simulink library "cbobsv2p5"  (Simulink 5.0)
values from neighbouring files (symbols this model uses):
  b = findobj(a, 'Name', get_param(gcbh,'Name'))    [eyediasi2.m]
undefined symbols (not defined in the file or in its folder): eyediasi2, remez
libraries: commblksprivate x14, dspsigattribs x10, dspmlti3 x6, simulink3 x6, dspsrcs4 x4, commsrccod2 x2, dsparch3 x1
settings Model: Creator=mmclerno  LastModifiedBy=mclune  ExtModeAutoUpdateStatusClock=off

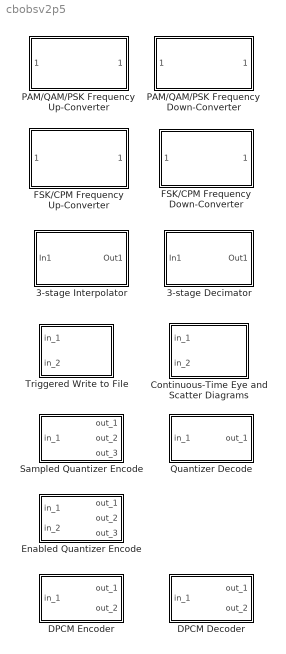
== system cbobsv2p5 ==
  3-stage Decimator : Subsystem  mask(3-stage Decimator){decFactor=10, Tin=1/10000, Fmax=450}
      mask prompts: decFactor "Decimation factor:"; Tin "Input sample time (s):"; Fmax "Maximum signal frequency (Hz):"
      mask help:
      | Performs decimation on the input signal.  The block uses multi-stage FIR filtering to eliminate aliasing, because using multiple stages is more efficient than using a single stage.
      |
      | For most efficient results, large decimation factors should have at least three factors.
      mask init:
      | dec_params = commblkdecimtr(gcb,'init');
      mask Display: disp('3-stage\nDecimator')
  3-stage Interpolator : Subsystem  mask(3-stage Interpolator){intFactor=10, Tin=1/1000, Fmax=450}
      mask prompts: intFactor "Interpolation factor:"; Tin "Input sample time (s):"; Fmax "Maximum signal frequency (Hz):"
      mask help:
      | Performs a interpolation on the input signal.  The block uses multi-stage FIR filtering to eliminate spectral copies because using multiple stages is more efficient than using a single stage.
      |
      | For most efficient results, large interpolation factors should have at least three factors.
      mask init:
      | int_params = commblkintrpltr(gcb,'init');
      mask Display: disp('3-stage\n Interpolator')
  Continuous-Time Eye and Scatter Diagrams : Subsystem  LoadFcn=eyediasi2([],[],[],'LoadBlock')  StartFcn=eyediasi2([],[],[],'Start')  StopFcn=eyediasi2([],[],[],'Stop')  mask(Continuous-Time Eye and Scatter Diagrams){time_range=1, time_offset=0, boundary=[-1.5 1.5], kept_length=5, diagram_type=Eye Diagram, eye_line=b-/r-, scatter_line=b., two_d_line=b-}
      mask prompts: time_range "Trace period:"; time_offset "Trace offset:"; boundary "Lower and upper bounds of diagram (2-element vector):"; kept_length "Number of saved traces:"; diagram_type "Diagram type:"; eye_line "Line type for eye diagram:"; scatter_line "Line type for scatter diagram:"; two_d_line "Line type for X-Y diagram:"
      mask help: Create an eye diagram with or without a scatter diagram or an X-Y diagram depending on Diagram type parameter. Use the trigger input to determine the decision time for the scatter plot.
      mask init:
      | [a,b]=trigicon(0,25,get_param(gcb,'orientation'),2);
      | x = [2 8 5 2 8 5 5 5];
      | y = [2 8 5 8 2 5 8 2];
      | [eStr outparams] = commblkeyescatcont(gcb,'init');
      | if(eStr .ecode ~= 0)
      |    error(eStr .emsg);
      | end
      settings: CopyFcn=eyediasi2([],[],[],'CopyBlock')  DeleteFcn=eyediasi2([],[],[],'DeleteBlock')  NameChangeFcn=eyediasi2([],[],[],'NameChange')
      mask Help: helpview(commbhelp)
      mask StyleString: edit,edit,edit,edit,popup(Eye Diagram|Scatter Diagram|Eye and Scatter Diagrams|X-Y Diagram|Eye and X-Y Diagrams),edit,edit,edit
      mask CallbackString: ||||commblkeyescatcont(gcb,'cbDiagram_type');|||
      mask Display: plot(0,0,100,100,[5 45 45 5 5 5 5+40*[0:1/15:1] 5+40*[1:-1/15:0] 5+40*[0:1/15:1] 5+40*[1:-1/15:0]], [35 35 95 95 35 65 sin([0:1/15:1]*pi)*25+65 sin(-[0:1/15:1]*pi)*25+65 sin([0:1/15:1]*pi)*17+65 sin(-[0:1/15:1]*pi)*18+65]*.95+3 ,a,b, NaN, NaN, x+50,y+37,x+50,y+52,x+50,y+67,x+50,y+82, x+62,y+37,x+62,y+52,x+62,y+67,x+62,y+82, x+73,y+37,x+73,y+52,x+73,y+67,x+73,y+82, x+85,y+37,x+85,y+52,x+85,y+67,x+85,y+82, [50 95 73 73 73],[65 65 65 35 95])
  DPCM Decoder : Subsystem  mask(DPCM Decoder){num=[0 .9963], den=1, codebook=[-.0848 -.029 .0298 .0853], sample_time=.1}
      mask prompts: num "Predictor numerator:"; den "Predictor denominator:"; codebook "Quantization codebook:"; sample_time "Sample time:"
      mask help:
      | Input the DPCM coded index. Output DPCM decodes to the 1st outport and quantization decode to the 2nd outport.
      |
      | The input must be a scalar signal.
      mask Help: helpview(commbhelp)
      mask Display: disp('DPCM\ndecoder')
  DPCM Encoder : Subsystem  mask(DPCM Encoder){num=[0 .9963], den=1, partition=[-.0569 .0004 .0576], codebook=[-.0848 -.029 .0298 .0853], sample_time=.1}
      mask prompts: num "Predictor numerator:"; den "Predictor denominator:"; partition "Quantization partition:"; codebook "Quantization codebook:"; sample_time "Sample time:"
      mask help:
      | Output the DPCM encoded index to the 1st outport and the quantization recovered value to the 2nd outport.
      |
      | The input must be a scalar signal.
      mask Help: helpview(commbhelp)
      mask Display: disp('DPCM\nencoder')
  Enabled Quantizer Encode : Subsystem  mask(Enabled Quantizer Encode){partition=[-.75 -.25 .25 .75], codebook=[-.825 -.5 0 .5 .825], n=2}
      mask prompts: partition "Quantization partition:"; codebook "Quantization codebook:"; n "Input signal vector length:"
      mask help:
      | Triggered by the 2nd input signal, this block quantizes an analog signal to (1) digital signal, (2) quantization value, and (3) distortion.
      |
      | The first input can be either a scalar, a sample-based vector, or a frame-based row vector.  Each vector element is processed independently.
      |
      | The trigger input must be a scalar.
      mask init:
      | [x,y]=trigicon(0,25,get_param(gcb,'orientation'),1);
      mask Help: helpview(commbhelp)
      mask Display: plot(0,0,100,100,x,y);disp('Quantizer')
  FSK/CPM Frequency Down-Converter : Subsystem  mask(FSK/CPM Frequency Down-Converter){modType=FSK, M=8, freqSep=100, td=1/100, Fc=3000, Ph=0, Tin=1/10000, Tout=1/1000}
      mask prompts: modType "Modulation type:"; M "M-ary number:"; freqSep "Frequency separation (Hz):"; td "Symbol period (s):"; Fc "Carrier frequency (Hz):"; Ph "Carrier phase (rad):"; Tin "Input sample time (s):"; Tout "Output sample time (s):"
      mask help:
      | The FSK/CPM Frequency Down-Converter translates the frequency of the passband input signal to complex baseband.  It also decimates the signal in order to prevent aliasing.
      |
      | The input signal must be a sample-based scalar.
      mask init:
      | Fmax = commblkfskdowncon(gcb,'init');
      mask StyleString: popup(FSK|CPM),edit,edit,edit,edit,edit,edit,edit
      mask CallbackString: commblkfskdowncon(gcb,'cbModType');|||||||
      mask Display: disp('FSK/CPM\nFrequency\nDown-Converter');
  FSK/CPM Frequency Up-Converter : Subsystem  mask(FSK/CPM Frequency Up-Converter){modType=FSK, M=8, freqSep=100, td=1/100, Fc=3000, Ph=0, Tin=1/1000, Tout=1/10000}
      mask prompts: modType "Modulation type:"; M "M-ary number:"; freqSep "Frequency separation (Hz):"; td "Symbol period (s):"; Fc "Carrier frequency (Hz):"; Ph "Carrier phase (rad):"; Tin "Input sample time (s):"; Tout "Output sample time (s):"
      mask help:
      | The FSK/CPM Frequency Up-Converter translates the frequency of the baseband input FSK or CPM signal to the carrier frequency.
      | It also interpolates the signal in order to prevent aliasing.
      |
      | The input signal must be a sample-based scalar.
      mask init:
      | Fmax = commblkfskupcon(gcb,'init');
      mask StyleString: popup(FSK|CPM),edit,edit,edit,edit,edit,edit,edit
      mask CallbackString: commblkfskupcon(gcb,'cbModType');|||||||
      mask Display: disp('FSK/CPM\nFrequency\nUp-Converter');
  PAM/QAM/PSK Frequency Down-Converter : Subsystem  mask(PAM/QAM/PSK Frequency Down-Converter){Fc=3000, Ph=0, Tin=1/8000, Tout=1/100}
      mask prompts: Fc "Carrier frequency (Hz):"; Ph "Carrier phase (rad):"; Tin "Input sample time:"; Tout "Output sample time:"
      mask help:
      | The PAM/QAM/PSK Frequency Down-Converter translates the frequency of the input signal to complex baseband.  It also decimates the signal to a lower sampling frequency.
      |
      | The input signal must be a sample-based scalar.
      mask init:
      | if (Tin>=1/(2*(Fc+1/Tout))) error('The reciprocal of the input sample time must be greater than twice the sum of the carrier frequency and the reciprocal of the output sample time.'); end;
      | 
      | if (Tout <= 1/Fc) error('The reciprocal of the output sample time must be less than the carrier frequency.'); end;
      | 
      | if (Tin>=Tout) error('The input sample time must be less than the output sample time.'); end;
      mask Display: disp('PAM/QAM/PSK\nFrequency\nDown-Converter');
  PAM/QAM/PSK Frequency Up-Converter : Subsystem  mask(PAM/QAM/PSK Frequency Up-Converter){Fc=3000, Ph=0, Tin=1/100, Tout=1/8000}
      mask prompts: Fc "Carrier frequency (Hz):"; Ph "Carrier phase (rad):"; Tin "Input sample time:"; Tout "Output sample time:"
      mask help:
      | The PAM/QAM/PSK Frequency Up-Converter translates the frequency of the baseband input signal to the carrier frequency.  It also resamples the signal to a higher sampling frequency.
      |
      | The input signal must be a sample-based scalar.
      mask init:
      | if (Tout>=1/(2*(Fc+1/Tin))) error('The reciprocal of the output sample time must be greater than twice the sum of the carrier frequency and the reciprocal of the input sample time.'); end;
      | 
      | if (Tin <= 1/Fc) error('The reciprocal of the input sample time must be less than the carrier frequency.'); end;
      | 
      | if (Tin<=Tout) error('The input sample time must be greater than the output sample time.'); end;
      mask Display: disp('PAM/QAM/PSK\nFrequency\nUp-Converter');
  Quantizer Decode : Subsystem  mask(Quantizer Decode){codebook=[-.825 -.5 0, .5 .825]}
      mask prompts: codebook "Quantization codebook:"
      mask help:
      | Output the value in the given codebook based on the input index value.
      |
      | The input can be either a scalar, a sample-based vector, or a frame-based row vector.  This block processes each vector element independently.
      mask Help: helpview(commbhelp)
      mask Display: disp('Quantizer\ndecode')
  Sampled Quantizer Encode : Subsystem  mask(Sampled Quantizer Encode){partition=[-.75 -.25 .25 .75], codebook=[-.825 -.5 0 .5 .825], n=2, sample_time=.1}
      mask prompts: partition "Quantization partition:"; codebook "Quantization codebook:"; n "Input signal vector length:"; sample_time "Sample time:"
      mask help:
      | Quantize an analog signal to (1) digital signal, (2) quantization value, and (3) distortion at every sample time point.
      |
      | The input can be either a scalar, a sample-based vector, or a frame-based row vector.  This block processes each vector element independently.
      mask Help: helpview(commbhelp)
      mask Display: disp('Scalar\nquantizer')
  Triggered Write to File : Subsystem  mask(Triggered Write to File){filename='untitled.dat', datatype=ASCII, dec=1, threshold=0.5}
      mask prompts: filename "File name (string, include extension):"; datatype "Data type:"; dec "Decimation:"; threshold "Threshold in detecting trigger signal:"
      mask help:
      | The rising edge of the signal from the 2nd port triggers the block to write another row into the specified file.
      |
      | Inputs must be sample-based.
      mask init:
      | [x,y]=trigicon(0,25,get_param(gcb,'orientation'),2);
      | nump = dec - 1;
      mask Help: helpview(commbhelp)
      mask StyleString: edit,popup(ASCII|binary|float|integer),edit,edit
      mask Display:
      | plot(0,0,100,100,100-[25 25 05 05 25 25 05 13 13 17 17 17 15 real(exp(j*pi*([0:20]/10+1/2)))*3.5+15 15 25 25 25+[0:1/30:1]*70],
      | [85 95 95 75 75 89 89 89 95 95 89 89 89 imag(exp(j*pi*([0:20]/10+1/2)))*3.5+85 89 89 85 -sin([0:1/30:1]*pi*2)*10+85]-15, x,y);disp('\n  Wt file')

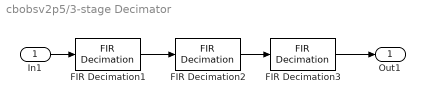
== system cbobsv2p5/3-stage Decimator ==
  In1 : Inport
  FIR Decimation1 : dspmlti3/FIR Decimation  h=remez(dec_params.order1, [0 dec_params.Fpass1 dec_params.Fstop1 1], [1 1 0 0])  D=dec_params.decFact1  framing=Maintain input frame size  outputBufInitCond=0
  FIR Decimation2 : dspmlti3/FIR Decimation  h=remez(dec_params.order2, [0 dec_params.Fpass2 dec_params.Fstop2 1], [1 1 0 0])  D=dec_params.decFact2  framing=Maintain input frame size  outputBufInitCond=0
  FIR Decimation3 : dspmlti3/FIR Decimation  h=remez(dec_params.order3, [0 dec_params.Fpass3 dec_params.Fstop3 1], [1 1 0 0])  D=dec_params.decFact3  framing=Maintain input frame size  outputBufInitCond=0
  Out1 : Outport
  wires:
  FIR Decimation1/1 -> FIR Decimation2/1
  FIR Decimation2/1 -> FIR Decimation3/1
  FIR Decimation3/1 -> Out1/1
  In1/1 -> FIR Decimation1/1

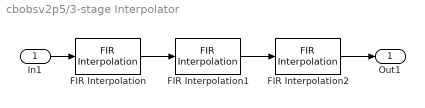
== system cbobsv2p5/3-stage Interpolator ==
  In1 : Inport
  FIR Interpolation : dspmlti3/FIR Interpolation  h=remez(int_params.order1, [0 int_params.Fpass1 int_params.Fstop1 1], [1 1 0 0]) * int_params.intFact1  L=int_params.intFact1  framing=Maintain input frame size  outputBufInitCond=0
  FIR Interpolation1 : dspmlti3/FIR Interpolation  h=remez(int_params.order2, [0 int_params.Fpass2 int_params.Fstop2 1], [1 1 0 0]) * int_params.intFact2  L=int_params.intFact2  framing=Maintain input frame size  outputBufInitCond=0
  FIR Interpolation2 : dspmlti3/FIR Interpolation  h=remez(int_params.order3, [0 int_params.Fpass3 int_params.Fstop3 1], [1 1 0 0]) * int_params.intFact3  L=int_params.intFact3  framing=Maintain input frame size  outputBufInitCond=0
  Out1 : Outport
  wires:
  FIR Interpolation2/1 -> Out1/1
  FIR Interpolation1/1 -> FIR Interpolation2/1
  FIR Interpolation/1 -> FIR Interpolation1/1
  In1/1 -> FIR Interpolation/1

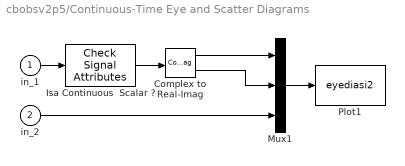
== system cbobsv2p5/Continuous-Time Eye and Scatter Diagrams ==
  in_1 : Inport
  in_2 : Inport  Port=2
  Complex to Real-Imag : ComplexToRealImag
  Isa Continuous  Scalar ? : dspsigattribs/Check Signal Attributes  SigAttribCheckMethod=Does not match attributes exactly  Complexity=Ignore  Frame=Sample-based  DimsCheckMethod=Is...  Dimensions=Scalar (1-D or 2-D)  DatatypeCheckMethod=Is not...  DatatypeGeneral=Boolean  DtypeFloatSpecific=Any floating-point  DtypeFixedSpecific=Any fixed-point  DtypeIntSpecific=Any integer  SampleMode=Continuous
  Mux1 : Mux  Inputs=3
  Plot1 : S-Function  FunctionName=eyediasi2  Parameters=time_range, time_offset, boundary, kept_length, diagram_type, eye_line, scatter_line, two_d_line
  wires:
  in_2/1 -> Mux1/3
  in_1/1 -> Isa Continuous  Scalar ?/1
  Complex to Real-Imag/2 -> Mux1/2
  Complex to Real-Imag/1 -> Mux1/1
  Mux1/1 -> Plot1/1
  Isa Continuous  Scalar ?/1 -> Complex to Real-Imag/1

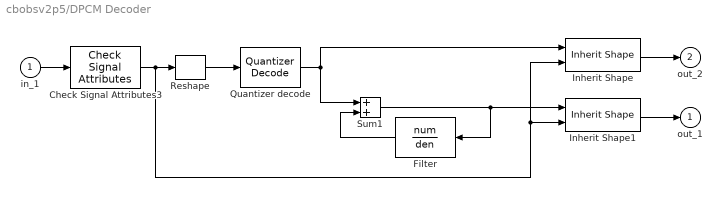
== system cbobsv2p5/DPCM Decoder ==
  in_1 : Inport
  Check Signal Attributes3 : dspsigattribs/Check Signal Attributes  SigAttribCheckMethod=Does not match attributes exactly  Complexity=Ignore  Frame=Ignore  DimsCheckMethod=Is...  Dimensions=Scalar (1-D or 2-D)  DatatypeCheckMethod=Ignore  DatatypeGeneral=Boolean  DtypeFloatSpecific=Any floating-point  DtypeFixedSpecific=Any fixed-point  DtypeIntSpecific=Any integer  SampleMode=Ignore
  Filter : DiscreteFilter  Orientation=left  Numerator=num  Denominator=den  SampleTime=sample_time
  Inherit Shape : commblksprivate/Inherit Shape
  Inherit Shape1 : commblksprivate/Inherit Shape
  Quantizer decode : commsrccod2/Quantizer Decode  codebook=codebook
  Reshape : simulink3/Signals & Systems/Reshape  OutputDimensionality=1-D array  OutputDimensions=[1,1]
  Sum1 : Sum  SaturateOnIntegerOverflow=on  InputSameDT=on
  out_1 : Outport  InitialOutput=0
  out_2 : Outport  Port=2  InitialOutput=0
  wires:
  Inherit Shape1/1 -> out_1/1
  Inherit Shape/1 -> out_2/1
  Reshape/1 -> Quantizer decode/1
  Check Signal Attributes3/1 -> Inherit Shape/2, Inherit Shape1/2, Reshape/1
  in_1/1 -> Check Signal Attributes3/1
  Filter/1 -> Sum1/2
  Sum1/1 -> Inherit Shape1/1, Filter/1
  Quantizer decode/1 -> Inherit Shape/1, Sum1/1

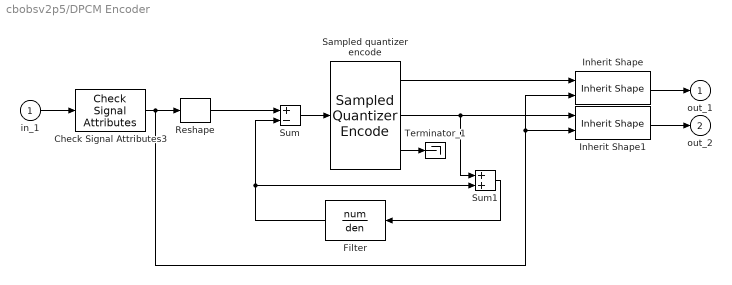
== system cbobsv2p5/DPCM Encoder ==
  in_1 : Inport
  Check Signal Attributes3 : dspsigattribs/Check Signal Attributes  SigAttribCheckMethod=Does not match attributes exactly  Complexity=Ignore  Frame=Ignore  DimsCheckMethod=Is...  Dimensions=Scalar (1-D or 2-D)  DatatypeCheckMethod=Ignore  DatatypeGeneral=Boolean  DtypeFloatSpecific=Any floating-point  DtypeFixedSpecific=Any fixed-point  DtypeIntSpecific=Any integer  SampleMode=Ignore
  Filter : DiscreteFilter  Orientation=left  Numerator=num  Denominator=den  SampleTime=sample_time
  Inherit Shape : commblksprivate/Inherit Shape
  Inherit Shape1 : commblksprivate/Inherit Shape
  Reshape : simulink3/Signals & Systems/Reshape  OutputDimensionality=1-D array  OutputDimensions=[1,1]
  Sampled quantizer encode : commsrccod2/Sampled Quantizer Encode  partition=partition  codebook=codebook  n=1  sample_time=sample_time
  Sum : Sum  Inputs=+-  SaturateOnIntegerOverflow=on  InputSameDT=on
  Sum1 : Sum  SaturateOnIntegerOverflow=on  InputSameDT=on
  Terminator_1 : Terminator
  out_1 : Outport  InitialOutput=0
  out_2 : Outport  Port=2  InitialOutput=0
  wires:
  Inherit Shape1/1 -> out_2/1
  Inherit Shape/1 -> out_1/1
  Sampled quantizer encode/1 -> Inherit Shape/1
  Reshape/1 -> Sum/1
  Check Signal Attributes3/1 -> Inherit Shape1/2, Inherit Shape/2, Reshape/1
  Sum1/1 -> Filter/1
  Filter/1 -> Sum/2, Sum1/2
  in_1/1 -> Check Signal Attributes3/1
  Sum/1 -> Sampled quantizer encode/1
  Sampled quantizer encode/2 -> Inherit Shape1/1, Sum1/1
  Sampled quantizer encode/3 -> Terminator_1/1

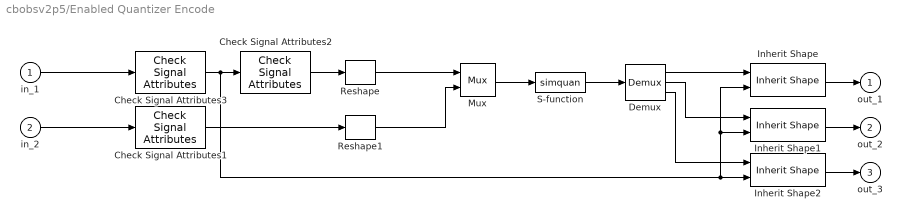
== system cbobsv2p5/Enabled Quantizer Encode ==
  in_1 : Inport
  in_2 : Inport  Port=2
  Check Signal Attributes1 : dspsigattribs/Check Signal Attributes  SigAttribCheckMethod=Does not match attributes exactly  Complexity=Ignore  Frame=Ignore  DimsCheckMethod=Is...  Dimensions=Scalar (1-D or 2-D)  DatatypeCheckMethod=Ignore  DatatypeGeneral=Boolean  DtypeFloatSpecific=Any floating-point  DtypeFixedSpecific=Any fixed-point  DtypeIntSpecific=Any integer  SampleMode=Ignore
  Check Signal Attributes2 : dspsigattribs/Check Signal Attributes  SigAttribCheckMethod=Matches attributes exactly  Complexity=Ignore  Frame=Frame-based  DimsCheckMethod=Is...  Dimensions=Column vector (2-D)  DatatypeCheckMethod=Ignore  DatatypeGeneral=Boolean  DtypeFloatSpecific=Any floating-point  DtypeFixedSpecific=Any fixed-point  DtypeIntSpecific=Any integer  SampleMode=Ignore
  Check Signal Attributes3 : dspsigattribs/Check Signal Attributes  SigAttribCheckMethod=Matches attributes exactly  Complexity=Ignore  Frame=Ignore  DimsCheckMethod=Is...  Dimensions=Full matrix (2-D)  DatatypeCheckMethod=Ignore  DatatypeGeneral=Boolean  DtypeFloatSpecific=Any floating-point  DtypeFixedSpecific=Any fixed-point  DtypeIntSpecific=Any integer  SampleMode=Ignore
  Demux : Demux  Outputs=[n n n]
  Inherit Shape : commblksprivate/Inherit Shape
  Inherit Shape1 : commblksprivate/Inherit Shape
  Inherit Shape2 : commblksprivate/Inherit Shape
  Mux : Mux  Inputs=[n 1]
  Reshape : simulink3/Signals & Systems/Reshape  OutputDimensionality=1-D array  OutputDimensions=[1,1]
  Reshape1 : simulink3/Signals & Systems/Reshape  OutputDimensionality=1-D array  OutputDimensions=[1,1]
  S-function : S-Function  FunctionName=simquan  Parameters=n, partition, codebook
  out_1 : Outport  InitialOutput=0
  out_2 : Outport  Port=2  InitialOutput=0
  out_3 : Outport  Port=3  InitialOutput=0
  wires:
  Reshape1/1 -> Mux/2
  Reshape/1 -> Mux/1
  Check Signal Attributes2/1 -> Reshape/1
  Check Signal Attributes1/1 -> Reshape1/1
  Demux/3 -> Inherit Shape2/1
  Demux/2 -> Inherit Shape1/1
  Inherit Shape2/1 -> out_3/1
  Inherit Shape1/1 -> out_2/1
  Demux/1 -> Inherit Shape/1
  Inherit Shape/1 -> out_1/1
  Check Signal Attributes3/1 -> Inherit Shape1/2, Inherit Shape/2, Inherit Shape2/2, Check Signal Attributes2/1
  in_1/1 -> Check Signal Attributes3/1
  in_2/1 -> Check Signal Attributes1/1
  Mux/1 -> S-function/1
  S-function/1 -> Demux/1

== system cbobsv2p5/FSK/CPM Frequency Down-Converter ==
  " " : Inport  SampleTime=Tin
  3-stage Decimator : commblksprivate/3-stage Decimator  decFactor=Tout / Tin  Tin=Tin  Fmax=Fmax
  Complex Carrier : dspsrcs4/Sine Wave  Amplitude=sqrt(2)  Frequency=-Fc  Phase=-Ph  SampleMode=Discrete  OutComplex=Complex  CompMethod=Trigonometric fcn  TableSize=Speed  SampleTime=Tin  SamplesPerFrame=1  dType=Double  ResetState=Restart at time zero
  Product1 : Product  SaturateOnIntegerOverflow=on  InputSameDT=on
  "  " : Outport
  wires:
  Product1/1 -> 3-stage Decimator/1
  Complex Carrier/1 -> Product1/2
  " "/1 -> Product1/1
  3-stage Decimator/1 -> "  "/1

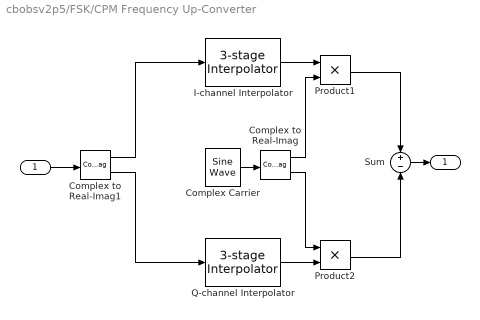
== system cbobsv2p5/FSK/CPM Frequency Up-Converter ==
  " " : Inport
  Complex Carrier : dspsrcs4/Sine Wave  Amplitude=sqrt(2)  Frequency=Fc  Phase=Ph  SampleMode=Discrete  OutComplex=Complex  CompMethod=Trigonometric fcn  TableSize=Speed  SampleTime=Tout  SamplesPerFrame=1  dType=Double  ResetState=Restart at time zero
  Complex to Real-Imag : ComplexToRealImag
  Complex to Real-Imag1 : ComplexToRealImag
  I-channel Interpolator : commblksprivate/3-stage Interpolator  intFactor=Tin / Tout  Tin=Tin  Fmax=Fmax
  Product1 : Product  SaturateOnIntegerOverflow=on  InputSameDT=on
  Product2 : Product  SaturateOnIntegerOverflow=on  InputSameDT=on
  Q-channel Interpolator : commblksprivate/3-stage Interpolator  intFactor=Tin / Tout  Tin=Tin  Fmax=Fmax
  Sum : Sum  Inputs=+|-  SaturateOnIntegerOverflow=on  InputSameDT=on
  "  " : Outport
  wires:
  Complex to Real-Imag1/1 -> I-channel Interpolator/1
  I-channel Interpolator/1 -> Product1/1
  Sum/1 -> "  "/1
  Product2/1 -> Sum/2
  Product1/1 -> Sum/1
  Complex to Real-Imag/2 -> Product2/1
  Complex to Real-Imag/1 -> Product1/2
  " "/1 -> Complex to Real-Imag1/1
  Complex Carrier/1 -> Complex to Real-Imag/1
  Q-channel Interpolator/1 -> Product2/2
  Complex to Real-Imag1/2 -> Q-channel Interpolator/1

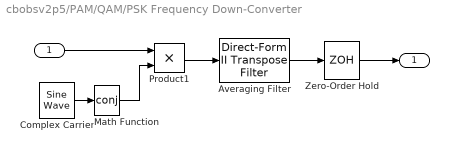
== system cbobsv2p5/PAM/QAM/PSK Frequency Down-Converter ==
  " " : Inport  SampleTime=Tin
  Averaging Filter : dsparch3/Direct-Form II Transpose Filter  num=(Tin/Tout)*ones(1,floor(Tout/Tin))  den=1  ic=0
  Complex Carrier : dspsrcs4/Sine Wave  Amplitude=sqrt(2)  Frequency=Fc  Phase=Ph  SampleMode=Discrete  OutComplex=Complex  CompMethod=Trigonometric fcn  TableSize=Speed  SampleTime=Tin  SamplesPerFrame=1  dType=Double  ResetState=Restart at time zero
  Math Function : Math  Operator=conj
  Product1 : Product  SaturateOnIntegerOverflow=on  InputSameDT=on
  Zero-Order Hold : ZeroOrderHold  SampleTime=Tout
  "  " : Outport
  wires:
  Averaging Filter/1 -> Zero-Order Hold/1
  Product1/1 -> Averaging Filter/1
  Complex Carrier/1 -> Math Function/1
  Math Function/1 -> Product1/2
  " "/1 -> Product1/1
  Zero-Order Hold/1 -> "  "/1

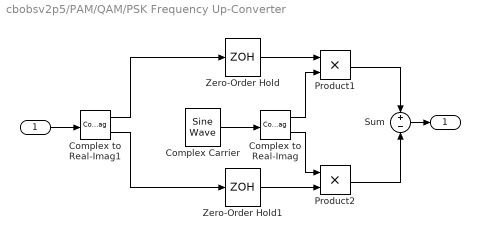
== system cbobsv2p5/PAM/QAM/PSK Frequency Up-Converter ==
  " " : Inport
  Complex Carrier : dspsrcs4/Sine Wave  Amplitude=sqrt(2)  Frequency=Fc  Phase=Ph  SampleMode=Discrete  OutComplex=Complex  CompMethod=Trigonometric fcn  TableSize=Speed  SampleTime=Tout  SamplesPerFrame=1  dType=Double  ResetState=Restart at time zero
  Complex to Real-Imag : ComplexToRealImag
  Complex to Real-Imag1 : ComplexToRealImag
  Product1 : Product  SaturateOnIntegerOverflow=on  InputSameDT=on
  Product2 : Product  SaturateOnIntegerOverflow=on  InputSameDT=on
  Sum : Sum  Inputs=+|-  SaturateOnIntegerOverflow=on  InputSameDT=on
  Zero-Order Hold : ZeroOrderHold  SampleTime=Tout
  Zero-Order Hold1 : ZeroOrderHold  SampleTime=Tout
  "  " : Outport
  wires:
  Complex Carrier/1 -> Complex to Real-Imag/1
  Sum/1 -> "  "/1
  Product2/1 -> Sum/2
  Product1/1 -> Sum/1
  Complex to Real-Imag/2 -> Product2/1
  Complex to Real-Imag/1 -> Product1/2
  Complex to Real-Imag1/1 -> Zero-Order Hold/1
  Complex to Real-Imag1/2 -> Zero-Order Hold1/1
  " "/1 -> Complex to Real-Imag1/1
  Zero-Order Hold/1 -> Product1/1
  Zero-Order Hold1/1 -> Product2/2

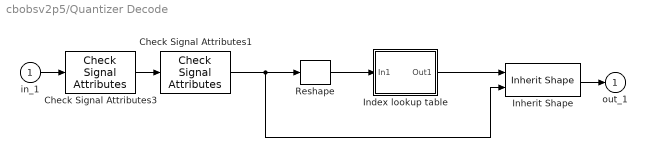
== system cbobsv2p5/Quantizer Decode ==
  in_1 : Inport
  Check Signal Attributes1 : dspsigattribs/Check Signal Attributes  SigAttribCheckMethod=Matches attributes exactly  Complexity=Ignore  Frame=Frame-based  DimsCheckMethod=Is...  Dimensions=Column vector (2-D)  DatatypeCheckMethod=Ignore  DatatypeGeneral=Boolean  DtypeFloatSpecific=Any floating-point  DtypeFixedSpecific=Any fixed-point  DtypeIntSpecific=Any integer  SampleMode=Ignore
  Check Signal Attributes3 : dspsigattribs/Check Signal Attributes  SigAttribCheckMethod=Matches attributes exactly  Complexity=Ignore  Frame=Ignore  DimsCheckMethod=Is...  Dimensions=Full matrix (2-D)  DatatypeCheckMethod=Ignore  DatatypeGeneral=Boolean  DtypeFloatSpecific=Any floating-point  DtypeFixedSpecific=Any fixed-point  DtypeIntSpecific=Any integer  SampleMode=Ignore
  Index lookup table : Subsystem  mask(No-intepret Lookup table){@1=codebook}
      mask prompts: @1 "Codebook:"
      mask help: Output one of the values in the look-up table.
      mask init:
      | codebook=@1;
      mask Help: When codebook is a matrix, the block input can only be a scalar. The block output the row with the column index provided in the input. When codebook is a vector, the block output the same length as the input vector. The output is one of the values in codebook with the index provided by the input.
      mask Display: disp('Index\nLookup tb')
  Inherit Shape : commblksprivate/Inherit Shape
  Reshape : simulink3/Signals & Systems/Reshape  OutputDimensionality=1-D array  OutputDimensions=[1,1]
  out_1 : Outport  InitialOutput=0
  wires:
  Check Signal Attributes1/1 -> Inherit Shape/2, Reshape/1
  Index lookup table/1(Out1) -> Inherit Shape/1
  Inherit Shape/1 -> out_1/1
  Reshape/1 -> Index lookup table/1(In1)
  Check Signal Attributes3/1 -> Check Signal Attributes1/1
  in_1/1 -> Check Signal Attributes3/1

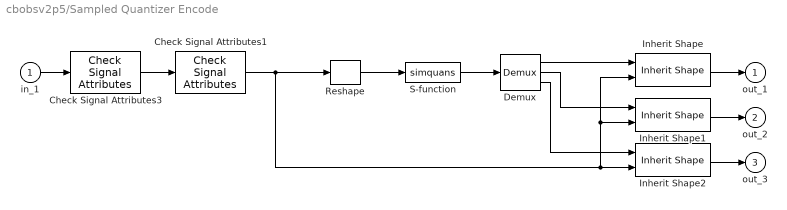
== system cbobsv2p5/Sampled Quantizer Encode ==
  in_1 : Inport
  Check Signal Attributes1 : dspsigattribs/Check Signal Attributes  SigAttribCheckMethod=Matches attributes exactly  Complexity=Ignore  Frame=Frame-based  DimsCheckMethod=Is...  Dimensions=Column vector (2-D)  DatatypeCheckMethod=Ignore  DatatypeGeneral=Boolean  DtypeFloatSpecific=Any floating-point  DtypeFixedSpecific=Any fixed-point  DtypeIntSpecific=Any integer  SampleMode=Ignore
  Check Signal Attributes3 : dspsigattribs/Check Signal Attributes  SigAttribCheckMethod=Matches attributes exactly  Complexity=Ignore  Frame=Ignore  DimsCheckMethod=Is...  Dimensions=Full matrix (2-D)  DatatypeCheckMethod=Ignore  DatatypeGeneral=Boolean  DtypeFloatSpecific=Any floating-point  DtypeFixedSpecific=Any fixed-point  DtypeIntSpecific=Any integer  SampleMode=Ignore
  Demux : Demux  Outputs=[n n n]
  Inherit Shape : commblksprivate/Inherit Shape
  Inherit Shape1 : commblksprivate/Inherit Shape
  Inherit Shape2 : commblksprivate/Inherit Shape
  Reshape : simulink3/Signals & Systems/Reshape  OutputDimensionality=1-D array  OutputDimensions=[1,1]
  S-function : S-Function  FunctionName=simquans  Parameters=n, partition, codebook,sample_time
  out_1 : Outport  InitialOutput=0
  out_2 : Outport  Port=2  InitialOutput=0
  out_3 : Outport  Port=3  InitialOutput=0
  wires:
  Inherit Shape2/1 -> out_3/1
  Inherit Shape1/1 -> out_2/1
  Inherit Shape/1 -> out_1/1
  Check Signal Attributes1/1 -> Inherit Shape/2, Inherit Shape1/2, Inherit Shape2/2, Reshape/1
  Reshape/1 -> S-function/1
  Demux/3 -> Inherit Shape2/1
  Demux/2 -> Inherit Shape1/1
  Demux/1 -> Inherit Shape/1
  Check Signal Attributes3/1 -> Check Signal Attributes1/1
  S-function/1 -> Demux/1
  in_1/1 -> Check Signal Attributes3/1

== system cbobsv2p5/Triggered Write to File ==
  in_1 : Inport
  in_2 : Inport  Port=2
  Mux : Mux  Inputs=2
  S-function : S-Function  FunctionName=swritfil  Parameters=filename, datatype, nump, threshold
  Terminator : Terminator
  wires:
  S-function/1 -> Terminator/1
  Mux/1 -> S-function/1
  in_1/1 -> Mux/1
  in_2/1 -> Mux/2

== system cbobsv2p5/Quantizer Decode/Index lookup table ==
  In1 : Inport
  Index lookup table : S-Function  FunctionName=indxtabl  Parameters=codebook
  Out1 : Outport  InitialOutput=0
  wires:
  Index lookup table/1 -> Out1/1
  In1/1 -> Index lookup table/1
